simulink model "HW02_template"  (R2022b)
settings: Solver=ode4  StartTime=0.0  StopTime=20  FixedStep=1e-3  RelTol=1e-3  EnableMultiTasking=on
values from neighbouring files (symbols this model uses):
  V_ref = 100/3.6    (= 27.7777777778)    [run_template.m]
undefined symbols (not defined in the file or in its folder): par
libraries: simulink x2, slpidlib x1
settings Model: Creator=bshyrokau  LastModifiedBy=murt
settings SolverCC: AlgebraicLoopSolver=TrustRegion
settings DataIOCC: SaveOutput=off  SignalLogging=off  DSMLogging=off  SaveTime=off  ReturnWorkspaceOutputs=off
settings OptimizationCC: LifeSpan=inf
settings DebuggingCC: UnconnectedInputMsg=warning  UnconnectedOutputMsg=warning  UnconnectedLineMsg=warning  AllowSymbolicDim=off  SFUnexpectedBacktrackingDiag=warning  SFNoUnconditionalDefaultTransitionDiag=warning  SFExecutionAtInitializationDiag=none  SFMachineParentedDataDiag=warning  ArithmeticOperatorsInVariantConditions=warning
settings ModelReferenceCC: EnableRefExpFcnMdlSchedulingChecks=on  PropagateSignalLabelsOutOfModel=off
settings SFSimCC: SimUseLocalCustomCode=off  CustomCodeUndefinedFunction=UseInterfaceOnly
settings RTWCC: RTWUseLocalCustomCode=off  DLArmComputeVersion=19.05
settings CodeAppCC: StateflowObjectComments=on
settings GRTTargetCC: TargetLangStandard=C89/C90 (ANSI)
settings ConfigComp: CovMetricSettings=dw  CovSaveCumulativeToWorkspaceVar=on  CovSaveSingleToWorkspaceVar=on  CovExternalEMLEnable=off

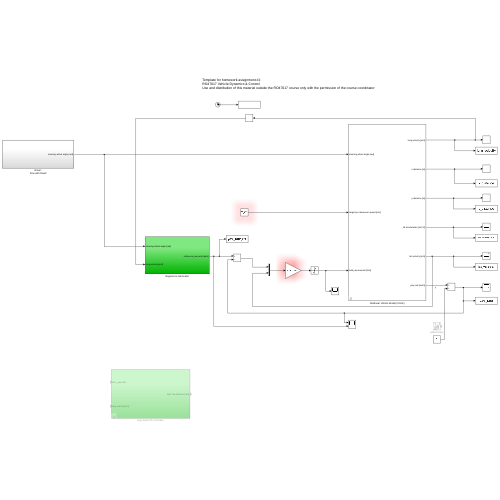
[thumbnail: Simulink's stored preview of the top-level diagram]
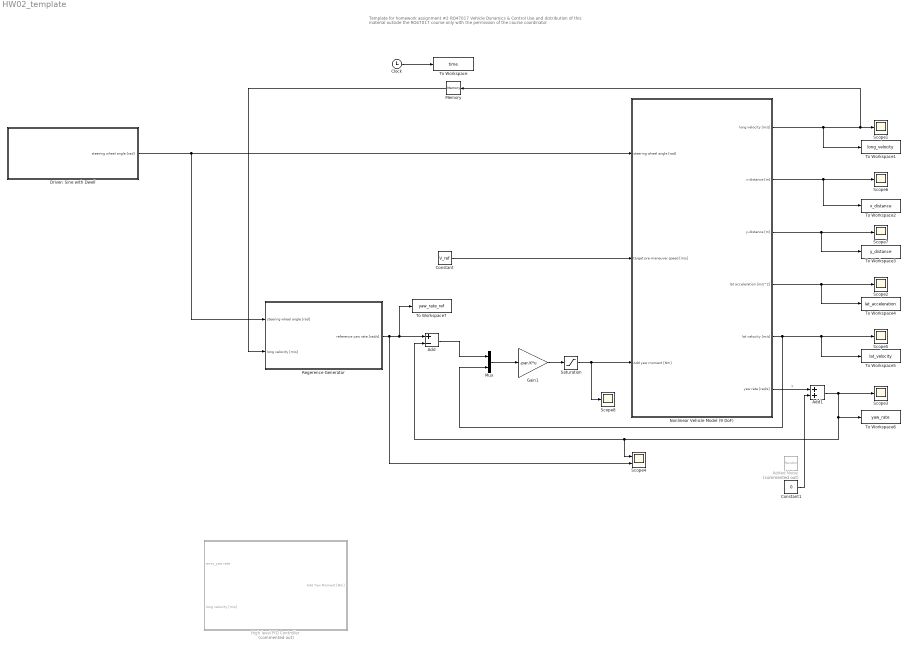
== system HW02_template ==
  note: Template for homework assignment #2
      | RO47017 Vehicle Dynamics & Control
      | Use and distribution of this material outside the RO47017 course only with the permission of the course coordinator
  Add : Sum  Inputs=+-
  Add1 : Sum
  Added Noise : UniformRandomNumber  Commented=on  Minimum=-0.01745/2  Maximum=0.01745/2
  Clock : Clock
  Constant : Constant  Value=V_ref
  Constant1 : Constant  Value=0
  Driver: Sine with Dwell : Subsystem
  Gain1 : Gain  Gain=-par.K*u
  High level PID Controller : Subsystem  Commented=on
  Memory : Memory
  Mux : Mux  Inputs=2
  Nonlinear Vehicle Model (9 DoF) : Subsystem
      mask help: Simulink:masks:GenSFuncDesc_MD
      mask Help: eval('feval(''rtwprivate'',''rtwhelpview'',''rtw_sfcn_block'')');
  Regerence Generator : Subsystem
  Saturation : Saturate  UpperLimit=10000  LowerLimit=-10000
  Scope{1..3,5..8} (7 alike) : Scope
  Scope4 : Scope  NumInputPorts=2
  To Workspace : ToWorkspace  VariableName=time  SampleTime=-1
  To Workspace1 : ToWorkspace  VariableName=long_velocity  SampleTime=-1
  To Workspace2 : ToWorkspace  VariableName=x_distance  SampleTime=-1
  To Workspace3 : ToWorkspace  VariableName=y_distance  SampleTime=-1
  To Workspace4 : ToWorkspace  VariableName=lat_acceleration  SampleTime=-1
  To Workspace5 : ToWorkspace  VariableName=lat_velocity  SampleTime=-1
  To Workspace6 : ToWorkspace  VariableName=yaw_rate  SampleTime=-1
  To Workspace7 : ToWorkspace  VariableName=yaw_rate_ref  SaveFormat=Timeseries  SampleTime=-1
  wires:
  Driver: Sine with Dwell/1(steering wheel angle [rad]) -> Nonlinear Vehicle Model (9 DoF)/1(steering wheel angle [rad]), Regerence Generator/1(steering wheel angle [rad])
  Regerence Generator/1(reference yaw rate [rad/s]) -> Scope4/2, To Workspace7/1, Add/1
  Nonlinear Vehicle Model (9 DoF)/1(long velocity [m/s]) -> To Workspace1/1, Memory/1, Scope1/1
  Nonlinear Vehicle Model (9 DoF)/4(lat acceleration [m/s^2]) -> To Workspace4/1, Scope2/1
  Nonlinear Vehicle Model (9 DoF)/2(x-distance [m]) -> To Workspace2/1, Scope6/1
  Nonlinear Vehicle Model (9 DoF)/3(y-distance [m]) -> To Workspace3/1, Scope7/1
  Constant/1 -> Nonlinear Vehicle Model (9 DoF)/2(target pre-maneuver speed [m/s])
  Clock/1 -> To Workspace/1
  Memory/1 -> Regerence Generator/2(long velocity [m/s])
  Nonlinear Vehicle Model (9 DoF)/6(yaw rate [rad/s]) -> Add1/1  "y"
  Constant1/1 -> Add1/2
  Add1/1 -> Scope3/1, Scope4/1, Add/2, To Workspace6/1
  Nonlinear Vehicle Model (9 DoF)/5(lat velocity [m/s]) -> Mux/2, To Workspace5/1, Scope5/1
  Gain1/1 -> Saturation/1
  Add/1 -> Mux/1
  Mux/1 -> Gain1/1
  Saturation/1 -> Scope8/1, Nonlinear Vehicle Model (9 DoF)/3(Add yaw moment [Nm])

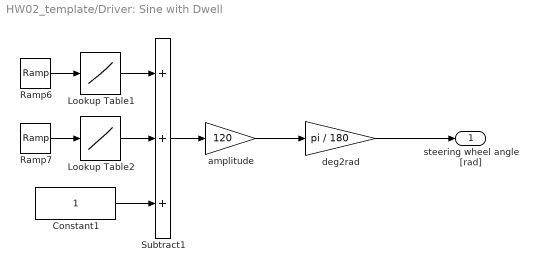
== system HW02_template/Driver: Sine with Dwell ==
  Constant1 : Constant
  Lookup Table1 : Lookup  InputValues=[0:0.1:3*pi/2 3*pi/2+eps]*0.7  Table=sin([0:0.1:3*pi/2 3*pi/2+eps])  LookUpMeth=Interpolation-Use End Values  SaturateOnIntegerOverflow=off
  Lookup Table2 : Lookup  InputValues=[3*pi/2:0.1:2*pi 2*pi+eps]*0.7  Table=sin([3*pi/2:0.1:2*pi 2*pi+eps])  LookUpMeth=Interpolation-Use End Values  SaturateOnIntegerOverflow=off
  Ramp6 : simulink/Sources/Ramp  slope=pi  start=10  InitialOutput=0
  Ramp7 : simulink/Sources/Ramp  slope=pi  start=10+0.5  InitialOutput=0
  Subtract1 : Sum  Inputs=+++
  amplitude : Gain  Gain=120
  deg2rad : Gain  Gain=pi / 180
  steering wheel angle [rad] : Outport  VectorParamsAs1DForOutWhenUnconnected=off
  wires:
  Ramp6/1 -> Lookup Table1/1
  Ramp7/1 -> Lookup Table2/1
  Lookup Table2/1 -> Subtract1/2
  Lookup Table1/1 -> Subtract1/1
  Constant1/1 -> Subtract1/3
  Subtract1/1 -> amplitude/1
  amplitude/1 -> deg2rad/1
  deg2rad/1 -> steering wheel angle [rad]/1

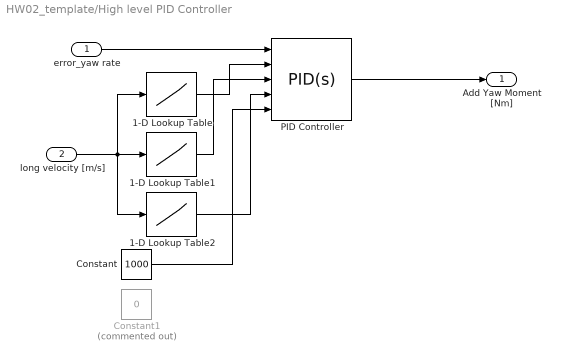
== system HW02_template/High level PID Controller ==
  error_yaw rate : Inport
  long velocity [m/s] : Inport  Port=2
  1-D Lookup Table : Lookup_n-D  NumberOfTableDimensions=1  BreakpointsForDimension1="[0   10   20   30]"  Table=[1000 10000 30000 50000]  InternalRulePriority=Speed  RndMeth=Simplest
  1-D Lookup Table1 : Lookup_n-D  NumberOfTableDimensions=1  BreakpointsForDimension1="[0   10   20   30]"  Table="[0  10  25  50]"  InternalRulePriority=Speed  RndMeth=Simplest
  1-D Lookup Table2 : Lookup_n-D  NumberOfTableDimensions=1  BreakpointsForDimension1="[0   10   20   30]"  Table="[10  20  50  100]"  InternalRulePriority=Speed  RndMeth=Simplest
  Constant : Constant  Value=1000
  Constant1 : Constant  Commented=on  Value=0
  PID Controller : slpidlib/PID Controller  Controller=PID  Form=Parallel  TimeDomain=Continuous-time  UseExternalTs=off  SampleTime=-1  IntegratorMethod=Forward Euler  FilterMethod=Forward Euler  ControllerParametersSource=external  P=50000  I=0  UseKiTs=off  D=10  N=1000  UseFilter=on  TunerSelectOption=Transfer Function Based (PID Tuner App)  InitialConditionSource=internal  InitialConditionForIntegrator=0  InitialConditionForFilter=0  DifferentiatorICPrevScaledInput=0  ExternalReset=none  TrackingMode=off  Kt=1  LimitOutput=off  SatLimitsSource=internal  UpperSaturationLimit=inf  LowerSaturationLimit=-inf  LinearizeAsGain=on  AntiWindupMode=none  Kb=1  LimitIntegrator=off  UpperIntegratorSaturationLimit=inf  LowerIntegratorSaturationLimit=-inf  POutMin=[]  POutMax=[]  IOutMin=[]  IOutMax=[]  DOutMin=[]  DOutMax=[]  NOutMin=[]  NOutMax=[]  SumOutMin=[]  SumOutMax=[]  SaturationOutMin=[]  SaturationOutMax=[]  PParamMin=[]  PParamMax=[]  IParamMin=[]  IParamMax=[]  DParamMin=[]  DParamMax=[]  NParamMin=[]  NParamMax=[]  KbParamMin=[]  KbParamMax=[]  KtParamMin=[]  KtParamMax=[]  KbOutMin=[]  KbOutMax=[]  KtOutMin=[]  KtOutMax=[]  IntegratorOutMin=[]  IntegratorOutMax=[]  FilterOutMin=[]  FilterOutMax=[]  SumI1OutMin=[]  SumI1OutMax=[]  SumI2OutMin=[]  SumI2OutMax=[]  SumI3OutMin=[]  SumI3OutMax=[]  SumI4OutMin=[]  SumI4OutMax=[]  SumDOutMin=[]  SumDOutMax=[]  DifferentiatorOutMin=[]  DifferentiatorOutMax=[]  FilterDiffOutCoefMin=[]  FilterDiffOutCoefMax=[]  ReciprocalOutMin=[]  ReciprocalOutMax=[]  SumDenOutMin=[]  SumDenOutMax=[]  SumNumOutMin=[]  SumNumOutMax=[]  DivideOutMin=[]  DivideOutMax=[]  UdiffTsProdOutMin=[]  UdiffTsProdOutMax=[]  NTsProdOutMin=[]  NTsProdOutMax=[]  UintegralTsProdOutMin=[]  UintegralTsProdOutMax=[]  UngainTsProdOutMin=[]  UngainTsProdOutMax=[]  ClampingZeroOutDataTypeStr=Inherit: Inherit via back propagation  ClampingZeroOutMin=[]  ClampingZeroOutMax=[]  FilterDenConstantOutDataTypeStr=Inherit: Inherit via back propagation  FilterDenConstantOutMin=[]  FilterDenConstantOutMax=[]  PCopyOutDataTypeStr=Inherit: Inherit via back propagation  PCopyOutMin=[]  PCopyOutMax=[]  NCopyOutDataTypeStr=Inherit: Inherit via back propagation  NCopyOutMin=[]  NCopyOutMax=[]  IntegratorContinuousStateAttributes=''  IntegratorStateMustResolveToSignalObject=off  IntegratorRTWStateStorageClass=Auto  FilterContinuousStateAttributes=''  FilterStateMustResolveToSignalObject=off  FilterRTWStateStorageClass=Auto  ParallelPVariant=ExternalParameters  IdealPVariant=Disabled  IVariant=ExternalParameters  DVariant=ExternalParameters  IntegratorVariant=Continuous  SatVariant=Disabled  AWVariant=Passthrough  PCopyVariant=Disabled  TRVariant=Disabled  FdbkBlocksVariant=Forward  IdealPFdbkVariant=Disabled  SatFdbkVariant=Disabled  DerivativeFilterVariant=ContFilter  NVariant=ExternalParameters  NCopyVariant=Disabled  FilterICVariant=InternalICsFilter  IntegratorICVariant=InternalICs  ExternalResetVariant=Disabled  TRSumVariant=Passthrough  SumFdbkVariant=Disabled  SumVariant=Sum_PID  TsampFilterVariant=InternalTs  TsampNgainVariant=Passthrough  TsampIntegralVariant=Passthrough  ExternalSaturationOutDataTypeStr=Inherit: Same as second input
  Add Yaw Moment [Nm] : Outport  VectorParamsAs1DForOutWhenUnconnected=off
  wires:
  error_yaw rate/1 -> PID Controller/1
  1-D Lookup Table/1 -> PID Controller/2
  long velocity [m/s]/1 -> 1-D Lookup Table/1, 1-D Lookup Table2/1, 1-D Lookup Table1/1
  1-D Lookup Table2/1 -> PID Controller/4
  Constant/1 -> PID Controller/5
  1-D Lookup Table1/1 -> PID Controller/3
  PID Controller/1 -> Add Yaw Moment [Nm]/1

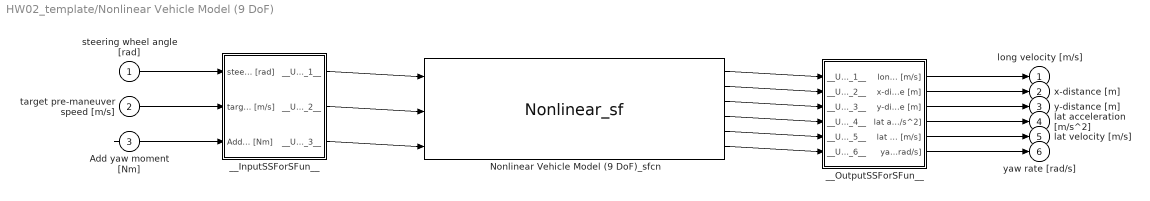
== system HW02_template/Nonlinear Vehicle Model (9 DoF) ==
  steering wheel angle [rad] : Inport
  target pre-maneuver speed [m/s] : Inport  Port=2
  Add yaw moment [Nm] : Inport  Port=3
  Nonlinear Vehicle Model (9 DoF)_sfcn : S-Function  FunctionName=Nonlinear_sf  SFunctionModules=""  SFunctionDeploymentMode=off  EnableBusSupport=off  mask{rtw_sf_name=Nonlinear_sf, showVar=off}
      mask prompts: rtw_sf_name "Simulink:masks:GenSFuncName_MP"; showVar "Simulink:masks:GenSFuncShowModuleList_MP"
      mask help: Simulink:masks:GenSFuncDesc_MD
      mask init:
      | displist = '';
      | if ~strcmp(get_param(gcb, 'FunctionName'), rtw_sf_name);
      |   set_param(gcb, 'FunctionName', rtw_sf_name);
      | end
      | % Check if we are generating code
      | rtw_mode = false;
      | if strcmpi(get_param(bdroot(gcb),'SimulationStatus'),'Initializing')
      | 	rtw_mode = strcmpi(get_param(bdroot(gcb),'BuildingRTWCode'),'on') && ...
      | 		~strcmpi(get_param(bdroot(gcb),'TargetStyle'),'SimulationTarget');
      | end
      | if showVar || rtw_mode
      | 	if exist('rtwsfunc') == 2 | exist('rtwsfunc') == 6
      | 		tmplist = rtwsfunc(rtw_sf_name,gcb);
      | 		tmplist = DAStudio.message('Simulink:masks:GenSFuncListOfModules_IC', tmplist);
      | 	elseif showVar
      | 		tmplist1 = DAStudio.message('Simulink:masks:GenSFuncListOfModules_IC', '');
      |         tmplist2 = DAStudio.message('Simulink:masks:GenSFuncNotLicensed_IC');
      |         tmplist = [tmplist1 tmplist2];
      |  	end
      | end
      | if showVar
      |   displist = tmplist;
      | end
      settings: CopyFcn=|
      | if ~strcmp(get_param(gcb,'Linkstatus'),'none') && ...
      | ~strcmp(get_param(gcb,'Linkstatus'),'implicit')
      |   set_param(gcb,'LinkStatus','none');
      | end
      mask Help: eval('feval(''rtwprivate'',''rtwhelpview'',''rtw_sfcn_block'')');
      mask Display:
      | port_label('input',1,'steering wheel angle [rad]');
      | port_label('input',2,'target pre-maneuver speed [m/s]');
      | port_label('input',3,'Add yaw moment [Nm]');
      | port_label('output',1,'long velocity [m/s]');
      | port_label('output',2,'x-distance [m]');
      | port_label('output',3,'y-distance [m]');
      | port_label('output',4,'lat acceleration [m/s^2]');
      | port_label('output',5,'lat velocity [m/s]');
      | port_label('output',6,'yaw rate [rad/s]');
  __InputSSForSFun__ : Subsystem
  __OutputSSForSFun__ : Subsystem
  long velocity [m/s] : Outport  VectorParamsAs1DForOutWhenUnconnected=off
  x-distance [m] : Outport  Port=2  VectorParamsAs1DForOutWhenUnconnected=off
  y-distance [m] : Outport  Port=3  VectorParamsAs1DForOutWhenUnconnected=off
  lat acceleration [m/s^2] : Outport  Port=4  VectorParamsAs1DForOutWhenUnconnected=off
  lat velocity [m/s] : Outport  Port=5  VectorParamsAs1DForOutWhenUnconnected=off
  yaw rate [rad/s] : Outport  Port=6  VectorParamsAs1DForOutWhenUnconnected=off
  wires:
  steering wheel angle [rad]/1 -> __InputSSForSFun__/1(steering wheel angle [rad])
  target pre-maneuver speed [m/s]/1 -> __InputSSForSFun__/2(target pre-maneuver speed [m/s])
  Add yaw moment [Nm]/1 -> __InputSSForSFun__/3(Add yaw moment [Nm])
  __InputSSForSFun__/1(__UniqueOutportName__1__) -> Nonlinear Vehicle Model (9 DoF)_sfcn/1
  __InputSSForSFun__/2(__UniqueOutportName__2__) -> Nonlinear Vehicle Model (9 DoF)_sfcn/2
  __InputSSForSFun__/3(__UniqueOutportName__3__) -> Nonlinear Vehicle Model (9 DoF)_sfcn/3
  Nonlinear Vehicle Model (9 DoF)_sfcn/1 -> __OutputSSForSFun__/1(__UniqueInportName__1__)
  Nonlinear Vehicle Model (9 DoF)_sfcn/2 -> __OutputSSForSFun__/2(__UniqueInportName__2__)
  Nonlinear Vehicle Model (9 DoF)_sfcn/3 -> __OutputSSForSFun__/3(__UniqueInportName__3__)
  Nonlinear Vehicle Model (9 DoF)_sfcn/4 -> __OutputSSForSFun__/4(__UniqueInportName__4__)
  Nonlinear Vehicle Model (9 DoF)_sfcn/5 -> __OutputSSForSFun__/5(__UniqueInportName__5__)
  Nonlinear Vehicle Model (9 DoF)_sfcn/6 -> __OutputSSForSFun__/6(__UniqueInportName__6__)
  __OutputSSForSFun__/1(long velocity [m/s]) -> long velocity [m/s]/1
  __OutputSSForSFun__/2(x-distance [m]) -> x-distance [m]/1
  __OutputSSForSFun__/3(y-distance [m]) -> y-distance [m]/1
  __OutputSSForSFun__/4(lat acceleration [m/s^2]) -> lat acceleration [m/s^2]/1
  __OutputSSForSFun__/5(lat velocity [m/s]) -> lat velocity [m/s]/1
  __OutputSSForSFun__/6(yaw rate [rad/s]) -> yaw rate [rad/s]/1

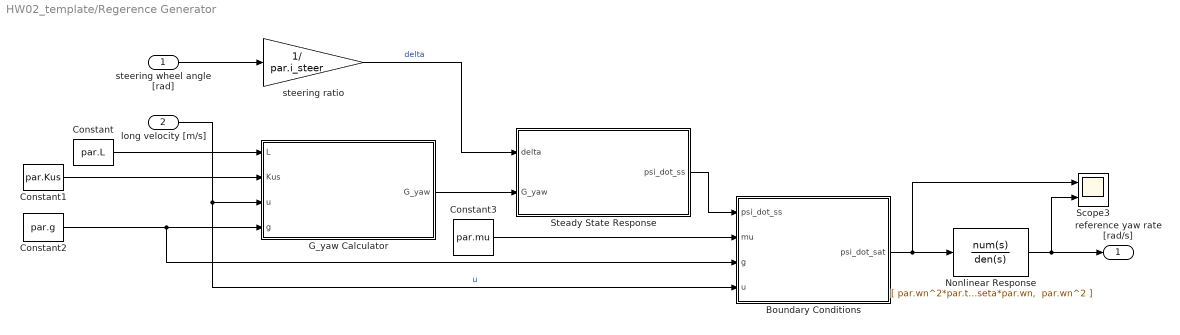
== system HW02_template/Regerence Generator ==
  steering wheel angle [rad] : Inport
  long velocity [m/s] : Inport  Port=2
  Boundary Conditions : MATLAB Function  TreatAsAtomicUnit=on
  Constant : Constant  Value=par.L
  Constant1 : Constant  Value=par.Kus
  Constant2 : Constant  Value=par.g
  Constant3 : Constant  Value=par.mu
  G_yaw Calculator : MATLAB Function  TreatAsAtomicUnit=on
  Nonlinear Response : TransferFcn  Numerator="[ par.wn^2*par.tau,  par.wn^2 ]"  Denominator="[ 1,  2*par.kseta*par.wn,  par.wn^2 ]"
  Scope3 : Scope  NumInputPorts=2
  Steady State Response : MATLAB Function  TreatAsAtomicUnit=on
  steering ratio : Gain  Gain=1/ par.i_steer
  reference yaw rate [rad/s] : Outport  VectorParamsAs1DForOutWhenUnconnected=off
  wires:
  Nonlinear Response/1 -> reference yaw rate [rad/s]/1, Scope3/2
  steering wheel angle [rad]/1 -> steering ratio/1
  steering ratio/1 -> Steady State Response/1(delta)  "delta"
  Boundary Conditions/1(psi_dot_sat) -> Nonlinear Response/1, Scope3/1
  Steady State Response/1(psi_dot_ss) -> Boundary Conditions/1(psi_dot_ss)
  long velocity [m/s]/1 -> G_yaw Calculator/3(u), Boundary Conditions/4(u)  "u"
  Constant/1 -> G_yaw Calculator/1(L)
  Constant2/1 -> Boundary Conditions/3(g), G_yaw Calculator/4(g)
  Constant1/1 -> G_yaw Calculator/2(Kus)
  G_yaw Calculator/1(G_yaw) -> Steady State Response/2(G_yaw)
  Constant3/1 -> Boundary Conditions/2(mu)

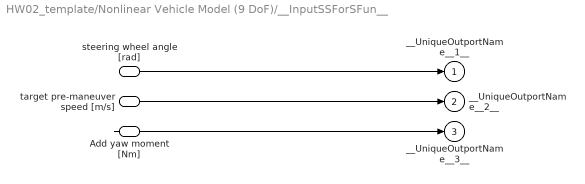
== system HW02_template/Nonlinear Vehicle Model (9 DoF)/__InputSSForSFun__ ==
  steering wheel angle [rad] : Inport
  target pre-maneuver speed [m/s] : Inport  Port=2
  Add yaw moment [Nm] : Inport  Port=3
  __UniqueOutportName__1__ : Outport
  __UniqueOutportName__2__ : Outport  Port=2
  __UniqueOutportName__3__ : Outport  Port=3
  wires:
  steering wheel angle [rad]/1 -> __UniqueOutportName__1__/1
  target pre-maneuver speed [m/s]/1 -> __UniqueOutportName__2__/1
  Add yaw moment [Nm]/1 -> __UniqueOutportName__3__/1

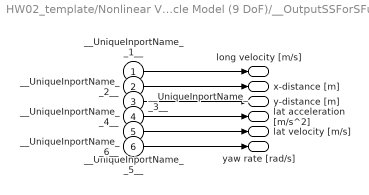
== system HW02_template/Nonlinear Vehicle Model (9 DoF)/__OutputSSForSFun__ ==
  __UniqueInportName__1__ : Inport
  __UniqueInportName__2__ : Inport  Port=2
  __UniqueInportName__3__ : Inport  Port=3
  __UniqueInportName__4__ : Inport  Port=4
  __UniqueInportName__5__ : Inport  Port=5
  __UniqueInportName__6__ : Inport  Port=6
  long velocity [m/s] : Outport  VectorParamsAs1DForOutWhenUnconnected=off
  x-distance [m] : Outport  Port=2  VectorParamsAs1DForOutWhenUnconnected=off
  y-distance [m] : Outport  Port=3  VectorParamsAs1DForOutWhenUnconnected=off
  lat acceleration [m/s^2] : Outport  Port=4  VectorParamsAs1DForOutWhenUnconnected=off
  lat velocity [m/s] : Outport  Port=5  VectorParamsAs1DForOutWhenUnconnected=off
  yaw rate [rad/s] : Outport  Port=6  VectorParamsAs1DForOutWhenUnconnected=off
  wires:
  __UniqueInportName__1__/1 -> long velocity [m/s]/1
  __UniqueInportName__2__/1 -> x-distance [m]/1
  __UniqueInportName__3__/1 -> y-distance [m]/1
  __UniqueInportName__4__/1 -> lat acceleration [m/s^2]/1
  __UniqueInportName__5__/1 -> lat velocity [m/s]/1
  __UniqueInportName__6__/1 -> yaw rate [rad/s]/1

== matlab function HW02_template/Regerence Generator/Steady State Response ==
  data: delta input; G_yaw input; psi_dot_ss output
function psi_dot_ss = SteadyStateResponse(delta, G_yaw)
  psi_dot_ss = G_yaw * delta;
end

== matlab function HW02_template/Regerence Generator/Boundary Conditions ==
  data: psi_dot_ss input; psi_dot_sat output; mu input; g input; u input
function psi_dot_sat = BoundaryConditions(psi_dot_ss, mu, g, u)
  % compute the maximum allowable yaw rate magnitude
  psi_dot_max = 0.85 * (mu * g) / u;

  % clamp psi_dot_ss to the interval [‑psi_dot_max, +psi_dot_max]
  if abs(psi_dot_ss) <= abs(psi_dot_max)
    % inside the limits → pass straight through
    psi_dot_sat = psi_dot_ss;
  else
    % outside the limits → saturate at ±psi_dot_max
    psi_dot_sat = sign(psi_dot_ss) * psi_dot_max;
  end
end

== matlab function HW02_template/Regerence Generator/G_yaw Calculator ==
  data: L input; Kus input; G_yaw output; u input; g input
function G_yaw = GyawCalculator(L, Kus, u, g)
  G_yaw     = u/(L + (Kus*u^2/g));
end
